simulink model "drone"  (R2022b)
settings: Solver=FixedStepDiscrete  StartTime=0.0  StopTime=0.1  FixedStep=0.01  RelTol=1e-3
settings Model: Creator=IvanRakov  LastModifiedBy=IvanRakov

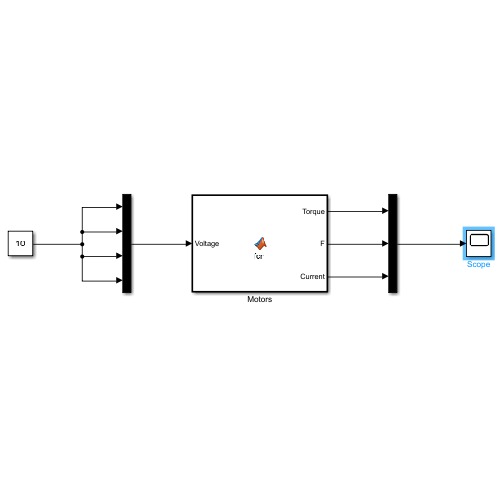
[thumbnail: Simulink's stored preview of the top-level diagram]
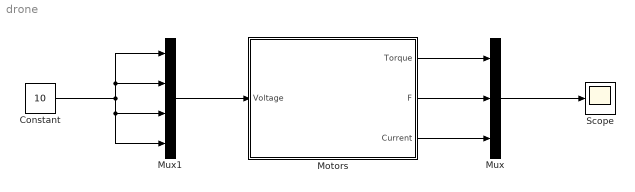
== system drone ==
  Constant : Constant  Value=10  SampleTime=0.01
  Motors : MATLAB Function  TreatAsAtomicUnit=on
  Mux : Mux  Inputs=3
  Mux1 : Mux
  Scope : Scope
  wires:
  Motors/3(Current) -> Mux/3
  Motors/2(F) -> Mux/2
  Motors/1(Torque) -> Mux/1
  Mux/1 -> Scope/1
  Constant/1 -> Mux1/1, Mux1/2, Mux1/4, Mux1/3
  Mux1/1 -> Motors/1(Voltage)

== matlab function drone/Motors ==
  data: Voltage input; Torque output; F output; Current output
function [Torque, F, Current] = fcn(Voltage)

RPM = [0 0 0 0];
Torque = [0 0 0 0];
F = [0 0 0 0];
Current = [0 0 0 0];

for i = 1:4
    RPM(i) = -2.6931*Voltage(i)^3 + 1400*Voltage(i);
    Ct = 2*10^-15 * RPM(i)^3 - 4*10^-11 * RPM(i)^2 + 3*10^-7 * RPM(i) + 0.10113;
    F(i) = Ct * 1.225 * (RPM(i)/60)^2 * 0.2^4;
    Torque(i) = 4*10^-14 * RPM(i)^3 + 8*10^-12 * RPM(i)^2 + 3*10^-6 * RPM(i);
    Current(i) = 1400 * Torque(i);
end
